simulink model "pi_OfflineRL_H2DF_2023a"  (R2023a)
settings: Solver=FixedStepAuto  StartTime=0.0  StopTime=inf  FixedStep=0.001  RelTol=1e-3  EnableMultiTasking=on
values from neighbouring files (symbols this model uses):
  C2C_NMPC = init_C2C_NMPC_H2DF(C2C_NMPC.expdata)    [init_pi_OfflineRL_H2DF_2023a.m]
  LowerLimit = ([0.17e-3;350;-2;2e-3] - C2C_NMPC.Normalization.controls.mean)./(C2C_NMPC.Normalization.controls.std)    [init_pi_OfflineRL_H2DF_2023a.m]
  UpperLimit = ([0.5e-3;900;10;5.5e-3] - C2C_NMPC.Normalization.controls.mean)./(C2C_NMPC.Normalization.controls.std)    [init_pi_OfflineRL_H2DF_2023a.m]
undefined symbols (not defined in the file or in its folder): DiscIntNeverNeededParam
libraries: deeplib x9, rllib x3, raspberrypiNetworklib x1
(part 2 of 4)

== system pi_OfflineRL_H2DF_2023a/main_C2C_RL/RL_Controller/State_Augmentation ==
  controls : Inport
  Delay1 : Delay  DelayLength=1  InitialCondition=C2C_NMPC.x0(1:C2C_NMPC.Dims.n_LSTM_states)
  Delay3 : Delay  DelayLength=1  InitialCondition=C2C_NMPC.x0
  Delay4 : Delay  DelayLength=1  InitialCondition=C2C_NMPC.x0((C2C_NMPC.Dims.n_states - C2C_NMPC.Dims.n_outputs + 1):C2C_NMPC.Dims.n_states)
  Denorm_plant_IMEP_ref1 : Subsystem
  Display1 : Display
  Mux2 : Mux  Inputs=2
  Mux3 : Mux  Inputs=2
  Selector1 : Selector  IndexOptions=Index vector (dialog)  Indices=[(C2C_NMPC.Dims.n_states - C2C_NMPC.Dims.n_outputs + 1):C2C_NMPC.Dims.n_states]  OutputSizes=1
  Selector3 : Selector  IndexOptions=Index vector (dialog)  Indices=[1]  OutputSizes=1
  dyn_H2DF : Subsystem
  dyn_H2DF_state_augmentation : Subsystem
  LSTM_states : Outport
  wires:
  Delay3/1 -> Selector1/1
  Delay1/1 -> dyn_H2DF/3(last_LSTM_states), dyn_H2DF_state_augmentation/1(last_LSTM_states)
  dyn_H2DF_state_augmentation/1(LSTM_states) -> LSTM_states/1, Delay1/1, Mux3/1
  Mux2/1 -> Mux3/2
  controls/1 -> dyn_H2DF/1(controls), [controls]
  Selector1/1 -> dyn_H2DF/2(last_outputs)
  [controls] -> dyn_H2DF_state_augmentation/2(controls), Mux2/1
  Delay4/1 -> dyn_H2DF_state_augmentation/3(last_outputs)
  Mux3/1 -> Delay3/1
  Denorm_plant_IMEP_ref1/1(RefIn) -> Display1/1
  Selector3/1 -> Denorm_plant_IMEP_ref1/1(outputs)
  dyn_H2DF/1(outputs) -> Selector3/1, Delay4/1, Mux2/2

== system pi_OfflineRL_H2DF_2023a/main_C2C_RL/RL_Controller/Subsystem ==
  note: SOOT
  note: NOX
  note: IMEP
  note: MPRR
  last_outputs : Inport
  Constant : Constant  Value=C2C_NMPC.Normalization.outputs.mean(1)
  Constant1 : Constant  Value=4.8e5
  Constant{4,7,10,12} (4 alike) : Constant  Value=0
  Constant2 : Constant  Value=C2C_NMPC.Normalization.outputs.mean(2)
  Constant3 : Constant  Value=280
  Constant5 : Constant  Value=C2C_NMPC.Normalization.outputs.mean(3)
  Constant6 : Constant  Value=0.1
  Constant8 : Constant  Value=C2C_NMPC.Normalization.outputs.mean(4)
  Constant9 : Constant  Value=5e5
  Demux : Demux
  Gain : Gain  Gain=1/C2C_NMPC.Normalization.outputs.std(1)
  Gain1 : Gain  Gain=1/C2C_NMPC.Normalization.outputs.std(2)
  Gain2 : Gain  Gain=1/C2C_NMPC.Normalization.outputs.std(3)
  Gain3 : Gain  Gain=1/C2C_NMPC.Normalization.outputs.std(4)
  Gain{4..7} (4 alike) : Gain
  Mux : Mux
  Sum{1..3,5} (4 alike) : Sum  Inputs=|+-
  Switch{,1..3} (4 alike) : Switch  Criteria=u2 > Threshold  SaturateOnIntegerOverflow=off  InputSameDT=off
  last_Outputs_Override : Outport
  wires:
  Demux/1 -> Gain4/1
  Constant12/1 -> Switch/2
  last_outputs/1 -> Demux/1
  Constant/1 -> Sum5/2
  Sum5/1 -> Gain/1
  Constant1/1 -> Sum5/1
  Gain/1 -> Switch/1
  Sum1/1 -> Gain1/1
  Constant2/1 -> Sum1/2
  Constant3/1 -> Sum1/1
  Constant4/1 -> Switch1/2
  Gain1/1 -> Switch1/1
  Demux/2 -> Gain5/1
  Switch1/1 -> Mux/2
  Switch2/1 -> Mux/3
  Constant6/1 -> Sum2/1
  Constant5/1 -> Sum2/2
  Sum2/1 -> Gain2/1
  Constant7/1 -> Switch2/2
  Demux/3 -> Gain6/1
  Gain2/1 -> Switch2/1
  Switch3/1 -> Mux/4
  Constant9/1 -> Sum3/1
  Constant8/1 -> Sum3/2
  Sum3/1 -> Gain3/1
  Constant10/1 -> Switch3/2
  Demux/4 -> Gain7/1
  Gain3/1 -> Switch3/1
  Switch/1 -> Mux/1
  Mux/1 -> last_Outputs_Override/1
  Gain4/1 -> Switch/3
  Gain5/1 -> Switch1/3
  Gain6/1 -> Switch2/3
  Gain7/1 -> Switch3/3

== system pi_OfflineRL_H2DF_2023a/main_C2C_RL/RL_Controller/Subsystem1 ==
  In1 : Inport
  If : If  IfExpression=u1 > 4.5e5
  If Action Subsystem : Subsystem  TreatAsAtomicUnit=on
  If Action Subsystem1 : Subsystem  TreatAsAtomicUnit=on
  Merge : Merge
  Out1 : Outport
  wires:
  If Action Subsystem1/1(Out1) -> Merge/2
  If/2 -> If Action Subsystem1/Action
  If/1 -> If Action Subsystem/Action
  In1/1 -> If/1
  Merge/1 -> Out1/1
  If Action Subsystem/1(Out1) -> Merge/1

== system pi_OfflineRL_H2DF_2023a/main_C2C_RL/RL_Controller/dyn_H2DF_state_augmentation ==
  last_LSTM_states : Inport
  controls : Inport  Port=2
  last_outputs : Inport  Port=3
  dyn_H2DF_state_augmentation : MATLAB Function  TreatAsAtomicUnit=on
  LSTM_states : Outport
  wires:
  dyn_H2DF_state_augmentation/1(LSTM_states) -> LSTM_states/1
  last_outputs/1 -> dyn_H2DF_state_augmentation/3(last_outputs)
  last_LSTM_states/1 -> dyn_H2DF_state_augmentation/1(last_LSTM_states)
  controls/1 -> dyn_H2DF_state_augmentation/2(controls)

== system pi_OfflineRL_H2DF_2023a/main_C2C_RL/post_processing/ denormalizing reference ==
  IMEP_norm : Inport
  NOX_norm : Inport  Port=2
  soot_norm : Inport  Port=3
  MPRR_norm : Inport  Port=4
  Constant : Constant  Value=C2C_NMPC.Normalization.outputs.mean(1)
  Constant1 : Constant  Value=C2C_NMPC.Normalization.outputs.mean(2)
  Constant2 : Constant  Value=C2C_NMPC.Normalization.outputs.mean(3)
  Constant3 : Constant  Value=C2C_NMPC.Normalization.outputs.mean(4)
  Gain : Gain  Gain=C2C_NMPC.Normalization.outputs.std(1)
  Gain1 : Gain  Gain=C2C_NMPC.Normalization.outputs.std(2)
  Gain2 : Gain  Gain=C2C_NMPC.Normalization.outputs.std(3)
  Gain3 : Gain  Gain=C2C_NMPC.Normalization.outputs.std(4)
  Sum{1..3,5} (4 alike) : Sum  Inputs=|++
  IMEP : Outport
  NOX : Outport  Port=2
  soot : Outport  Port=3
  MPRR : Outport  Port=4
  wires:
  Gain/1 -> Sum5/1
  IMEP_norm/1 -> Gain/1
  Constant/1 -> Sum5/2
  Sum5/1 -> IMEP/1
  Gain1/1 -> Sum1/1
  Constant1/1 -> Sum1/2
  NOX_norm/1 -> Gain1/1
  Sum1/1 -> NOX/1
  Gain2/1 -> Sum2/1
  Constant2/1 -> Sum2/2
  soot_norm/1 -> Gain2/1
  Sum2/1 -> soot/1
  Gain3/1 -> Sum3/1
  Constant3/1 -> Sum3/2
  MPRR_norm/1 -> Gain3/1
  Sum3/1 -> MPRR/1

== system pi_OfflineRL_H2DF_2023a/main_C2C_RL/post_processing/Subsystem ==
  controller_ status : Inport
  LSTM_States : Inport  Port=2
  Selector2 : Selector  IndexOptions=Index vector (dialog)  Indices=[1:(C2C_NMPC.Dims.n_hidden_states+ C2C_NMPC.Dims.n_cell_states)]  OutputSizes=1
  Selector3 : Selector  IndexOptions=Index vector (dialog)  Indices=[41:56]  OutputSizes=1
  Subtract : Sum  Inputs=+-
  Out1 : Outport
  wires:
  Selector3/1 -> Subtract/1
  Selector2/1 -> Subtract/2
  controller_ status/1 -> Selector3/1
  Subtract/1 -> Out1/1
  LSTM_States/1 -> Selector2/1

== system pi_OfflineRL_H2DF_2023a/main_C2C_RL/post_processing/Subsystem1 ==
  controller_ status : Inport
  Last_Output_MC : Inport  Port=2
  " denormalizing reference" : Subsystem
  Demux : Demux
  Mux : Mux
  Mux1 : Mux  Inputs=2
  Mux2 : Mux
  Selector1 : Selector  IndexOptions=Index vector (dialog)  Indices=[(4 + C2C_NMPC.Dims.n_controls * C2C_NMPC.Opts.N + 1 * (C2C_NMPC.Dims.n_states) + C2C_NMPC.Dims.n_LSTM_states + C2C_NMPC.Dims.n_controls +1):( 4 + C2C_NMPC.Dims.n_controls * C2C_NMPC.Opts.N + 2* C2C_NMPC.Dims.n_states)]  OutputSizes=1
  Selector2 : Selector  IndexOptions=Index vector (dialog)  Indices=[(4 + C2C_NMPC.Dims.n_controls * C2C_NMPC.Opts.N + 2 * (C2C_NMPC.Dims.n_states) + C2C_NMPC.Dims.n_LSTM_states + C2C_NMPC.Dims.n_controls +1):( 4 + C2C_NMPC.Dims.n_controls * C2C_NMPC.Opts.N + 3* C2C_NMPC.Dims.n_states)]  OutputSizes=1
  Selector3 : Selector  IndexOptions=Index vector (dialog)  Indices=[(4 + C2C_NMPC.Dims.n_controls * C2C_NMPC.Opts.N + 1* (C2C_NMPC.Dims.n_LSTM_states + C2C_NMPC.Dims.n_controls) +1) : (4 + C2C_NMPC.Dims.n_controls * C2C_NMPC.Opts.N + 1* C2C_NMPC.Dims.n_states)]  OutputSizes=1
  Selector4 : Selector  IndexOptions=Index vector (dialog)  Indices=[(4 + C2C_NMPC.Dims.n_controls * C2C_NMPC.Opts.N + 3 * (C2C_NMPC.Dims.n_states) + C2C_NMPC.Dims.n_LSTM_states + C2C_NMPC.Dims.n_controls +1):( 4 + C2C_NMPC.Dims.n_controls * C2C_NMPC.Opts.N + 4* C2C_NMPC.Dims.n_states)]  OutputSizes=1
  Subsystem : Subsystem
  Out1 : Outport
  wires:
  Last_Output_MC/1 -> Demux/1
  controller_ status/1 -> Selector4/1, Selector2/1, Selector1/1, Selector3/1
  Mux1/1 -> Out1/1
  Mux/1 -> Mux1/2
  Demux/1 -> " denormalizing reference"/1(IMEP_norm)
  Demux/2 -> " denormalizing reference"/2(NOX_norm)
  Demux/3 -> " denormalizing reference"/3(soot_norm)
  Demux/4 -> " denormalizing reference"/4(MPRR_norm)
  " denormalizing reference"/2(NOX) -> Mux2/2
  " denormalizing reference"/1(IMEP) -> Mux2/1
  " denormalizing reference"/3(soot) -> Mux2/3
  " denormalizing reference"/4(MPRR) -> Mux2/4
  Mux2/1 -> Mux1/1
  Subsystem/1(Node_0) -> Mux/1
  Selector3/1 -> Subsystem/1(In1)
  Selector1/1 -> Subsystem/2(In2)
  Subsystem/2(Node_1) -> Mux/2
  Subsystem/3(Node_2) -> Mux/3
  Subsystem/4(Node_3) -> Mux/4
  Selector4/1 -> Subsystem/4(In4)
  Selector2/1 -> Subsystem/3(In3)

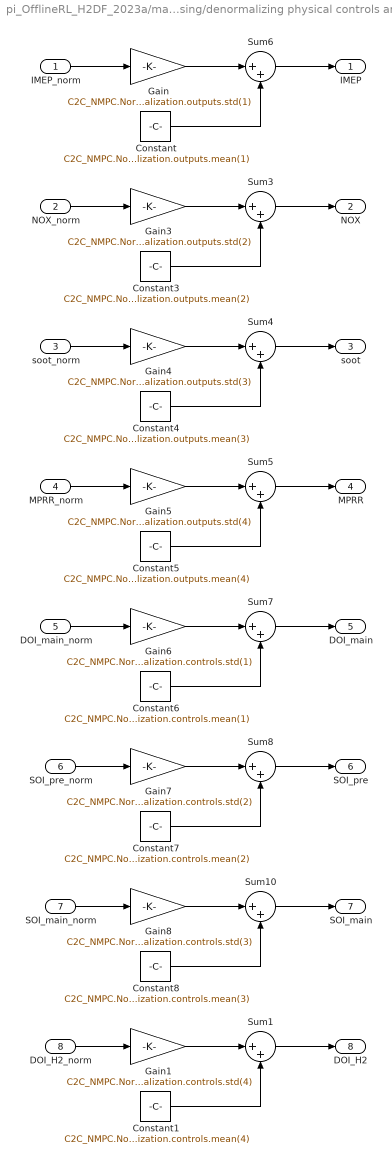
== system pi_OfflineRL_H2DF_2023a/main_C2C_RL/post_processing/denormalizing physical controls and outputs ==
  IMEP_norm : Inport
  NOX_norm : Inport  Port=2
  soot_norm : Inport  Port=3
  MPRR_norm : Inport  Port=4
  DOI_main_norm : Inport  Port=5
  SOI_pre_norm : Inport  Port=6
  SOI_main_norm : Inport  Port=7
  DOI_H2_norm : Inport  Port=8
  Constant : Constant  Value=C2C_NMPC.Normalization.outputs.mean(1)
  Constant1 : Constant  Value=C2C_NMPC.Normalization.controls.mean(4)
  Constant3 : Constant  Value=C2C_NMPC.Normalization.outputs.mean(2)
  Constant4 : Constant  Value=C2C_NMPC.Normalization.outputs.mean(3)
  Constant5 : Constant  Value=C2C_NMPC.Normalization.outputs.mean(4)
  Constant6 : Constant  Value=C2C_NMPC.Normalization.controls.mean(1)
  Constant7 : Constant  Value=C2C_NMPC.Normalization.controls.mean(2)
  Constant8 : Constant  Value=C2C_NMPC.Normalization.controls.mean(3)
  Gain : Gain  Gain=C2C_NMPC.Normalization.outputs.std(1)
  Gain1 : Gain  Gain=C2C_NMPC.Normalization.controls.std(4)
  Gain3 : Gain  Gain=C2C_NMPC.Normalization.outputs.std(2)
  Gain4 : Gain  Gain=C2C_NMPC.Normalization.outputs.std(3)
  Gain5 : Gain  Gain=C2C_NMPC.Normalization.outputs.std(4)
  Gain6 : Gain  Gain=C2C_NMPC.Normalization.controls.std(1)
  Gain7 : Gain  Gain=C2C_NMPC.Normalization.controls.std(2)
  Gain8 : Gain  Gain=C2C_NMPC.Normalization.controls.std(3)
  Sum{1,3..8,10} (8 alike) : Sum  Inputs=|++
  IMEP : Outport
  NOX : Outport  Port=2
  soot : Outport  Port=3
  MPRR : Outport  Port=4
  DOI_main : Outport  Port=5
  SOI_pre : Outport  Port=6
  SOI_main : Outport  Port=7
  DOI_H2 : Outport  Port=8
  wires:
  Gain4/1 -> Sum4/1
  Constant3/1 -> Sum3/2
  Constant4/1 -> Sum4/2
  Gain3/1 -> Sum3/1
  Constant5/1 -> Sum5/2
  Gain5/1 -> Sum5/1
  Constant/1 -> Sum6/2
  Sum3/1 -> NOX/1
  NOX_norm/1 -> Gain3/1
  Sum5/1 -> MPRR/1
  Gain/1 -> Sum6/1
  IMEP_norm/1 -> Gain/1
  Sum6/1 -> IMEP/1
  MPRR_norm/1 -> Gain5/1
  Sum4/1 -> soot/1
  soot_norm/1 -> Gain4/1
  Constant7/1 -> Sum8/2
  Gain8/1 -> Sum10/1
  Constant6/1 -> Sum7/2
  Gain7/1 -> Sum8/1
  Sum10/1 -> SOI_main/1
  DOI_main_norm/1 -> Gain6/1
  Sum7/1 -> DOI_main/1
  Gain6/1 -> Sum7/1
  Sum8/1 -> SOI_pre/1
  Constant8/1 -> Sum10/2
  SOI_main_norm/1 -> Gain8/1
  SOI_pre_norm/1 -> Gain7/1
  Sum1/1 -> DOI_H2/1
  Constant1/1 -> Sum1/2
  Gain1/1 -> Sum1/1
  DOI_H2_norm/1 -> Gain1/1

== system pi_OfflineRL_H2DF_2023a/main_C2C_RL/pre_processing1/normalize_last_outputs_MC ==
  data_in : Inport
  Constant : Constant  Value=C2C_NMPC.Normalization.outputs.mean(1)
  Constant1 : Constant  Value=C2C_NMPC.Normalization.outputs.mean(2)
  Constant2 : Constant  Value=C2C_NMPC.Normalization.outputs.mean(3)
  Constant3 : Constant  Value=C2C_NMPC.Normalization.outputs.mean(4)
  Demux : Demux
  Gain : Gain  Gain=1/C2C_NMPC.Normalization.outputs.std(1)
  Gain1 : Gain  Gain=1/C2C_NMPC.Normalization.outputs.std(2)
  Gain2 : Gain  Gain=1/C2C_NMPC.Normalization.outputs.std(3)
  Gain3 : Gain  Gain=1/C2C_NMPC.Normalization.outputs.std(4)
  Mux : Mux
  Selector1 : Selector  IndexOptions=Index vector (dialog)  Indices=[1:4]  OutputSizes=1
  Sum{1..3,5} (4 alike) : Sum  Inputs=|+-
  last_outputs_MC : Outport  VectorParamsAs1DForOutWhenUnconnected=off
  wires:
  Demux/2 -> Sum1/1
  Constant2/1 -> Sum2/2
  Sum2/1 -> Gain2/1
  Sum1/1 -> Gain1/1
  Gain3/1 -> Mux/4
  Gain1/1 -> Mux/2
  Constant1/1 -> Sum1/2
  Demux/3 -> Sum2/1
  Gain2/1 -> Mux/3
  Mux/1 -> last_outputs_MC/1
  Constant3/1 -> Sum3/2
  Sum3/1 -> Gain3/1
  Gain/1 -> Mux/1
  Sum5/1 -> Gain/1
  Constant/1 -> Sum5/2
  Demux/1 -> Sum5/1
  data_in/1 -> Selector1/1
  Demux/4 -> Sum3/1
  Selector1/1 -> Demux/1

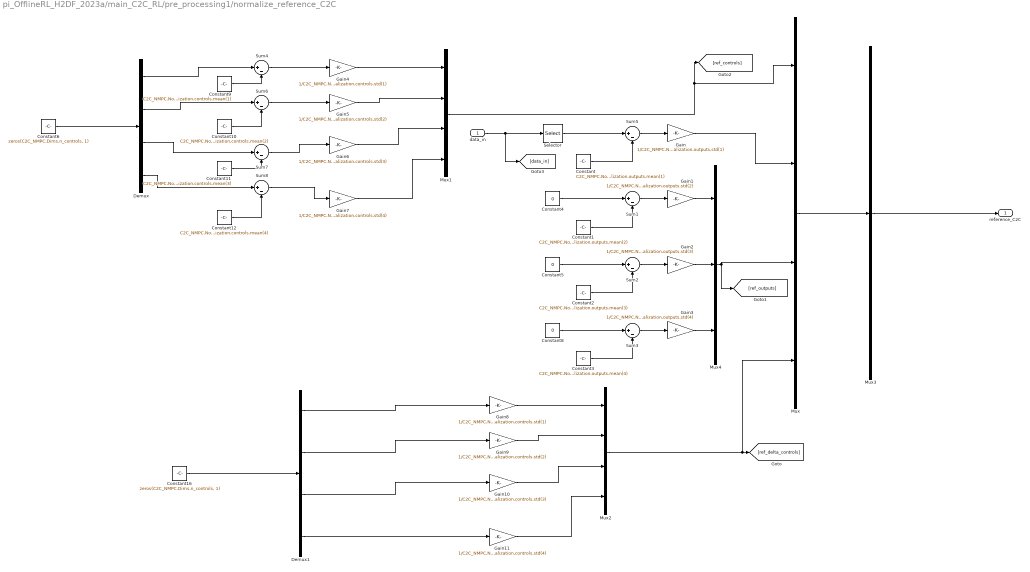
== system pi_OfflineRL_H2DF_2023a/main_C2C_RL/pre_processing1/normalize_reference_C2C ==
  data_in : Inport
  Constant : Constant  Value=C2C_NMPC.Normalization.outputs.mean(1)
  Constant1 : Constant  Value=C2C_NMPC.Normalization.outputs.mean(2)
  Constant10 : Constant  Value=C2C_NMPC.Normalization.controls.mean(2)
  Constant11 : Constant  Value=C2C_NMPC.Normalization.controls.mean(3)
  Constant12 : Constant  Value=C2C_NMPC.Normalization.controls.mean(4)
  Constant16 : Constant  Value=zeros(C2C_NMPC.Dims.n_controls, 1)
  Constant2 : Constant  Value=C2C_NMPC.Normalization.outputs.mean(3)
  Constant3 : Constant  Value=C2C_NMPC.Normalization.outputs.mean(4)
  Constant4 : Constant  Value=0
  Constant5 : Constant  Value=0
  Constant6 : Constant  Value=zeros(C2C_NMPC.Dims.n_controls, 1)
  Constant8 : Constant  Value=0
  Constant9 : Constant  Value=C2C_NMPC.Normalization.controls.mean(1)
  Demux : Demux
  Demux1 : Demux
  Gain : Gain  Gain=1/C2C_NMPC.Normalization.outputs.std(1)
  Gain1 : Gain  Gain=1/C2C_NMPC.Normalization.outputs.std(2)
  Gain10 : Gain  Gain=1/C2C_NMPC.Normalization.controls.std(3)
  Gain11 : Gain  Gain=1/C2C_NMPC.Normalization.controls.std(4)
  Gain2 : Gain  Gain=1/C2C_NMPC.Normalization.outputs.std(3)
  Gain3 : Gain  Gain=1/C2C_NMPC.Normalization.outputs.std(4)
  Gain4 : Gain  Gain=1/C2C_NMPC.Normalization.controls.std(1)
  Gain5 : Gain  Gain=1/C2C_NMPC.Normalization.controls.std(2)
  Gain6 : Gain  Gain=1/C2C_NMPC.Normalization.controls.std(3)
  Gain7 : Gain  Gain=1/C2C_NMPC.Normalization.controls.std(4)
  Gain8 : Gain  Gain=1/C2C_NMPC.Normalization.controls.std(1)
  Gain9 : Gain  Gain=1/C2C_NMPC.Normalization.controls.std(2)
  Mux : Mux
  Mux1 : Mux
  Mux2 : Mux
  Mux3 : Mux  Inputs=1
  Mux4 : Mux  Inputs=3
  Selector : Selector  IndexOptions=Index vector (dialog)  Indices=[5]  OutputSizes=1
  Sum{1..8} (8 alike) : Sum  Inputs=|+-
  reference_C2C : Outport  VectorParamsAs1DForOutWhenUnconnected=off
  wires:
  Constant/1 -> Sum5/2
  data_in/1 -> [data_in], Selector/1
  Sum5/1 -> Gain/1
  Selector/1 -> Sum5/1
  Constant4/1 -> Sum1/1
  Sum1/1 -> Gain1/1
  Constant1/1 -> Sum1/2
  Constant5/1 -> Sum2/1
  Sum2/1 -> Gain2/1
  Constant2/1 -> Sum2/2
  Constant8/1 -> Sum3/1
  Sum3/1 -> Gain3/1
  Constant3/1 -> Sum3/2
  Demux/1 -> Sum4/1
  Sum4/1 -> Gain4/1
  Constant9/1 -> Sum4/2
  Constant6/1 -> Demux/1
  Demux/2 -> Sum6/1
  Constant10/1 -> Sum6/2
  Sum6/1 -> Gain5/1
  Gain5/1 -> Mux1/2
  Gain4/1 -> Mux1/1
  Sum7/1 -> Gain6/1
  Constant11/1 -> Sum7/2
  Demux/3 -> Sum7/1
  Constant12/1 -> Sum8/2
  Sum8/1 -> Gain7/1
  Demux/4 -> Sum8/1
  Gain7/1 -> Mux1/4
  Gain6/1 -> Mux1/3
  Gain9/1 -> Mux2/2
  Gain11/1 -> Mux2/4
  Constant16/1 -> Demux1/1
  Gain8/1 -> Mux2/1
  Gain10/1 -> Mux2/3
  Demux1/4 -> Gain11/1
  Demux1/3 -> Gain10/1
  Demux1/2 -> Gain9/1
  Demux1/1 -> Gain8/1
  Mux2/1 -> [ref_delta_controls], Mux/4
  Mux3/1 -> reference_C2C/1
  Mux/1 -> Mux3/1
  Gain1/1 -> Mux4/1
  Gain2/1 -> Mux4/2
  Gain3/1 -> Mux4/3
  Gain/1 -> Mux/2
  Mux4/1 -> Mux/3, [ref_outputs]
  Mux1/1 -> [ref_controls], Mux/1

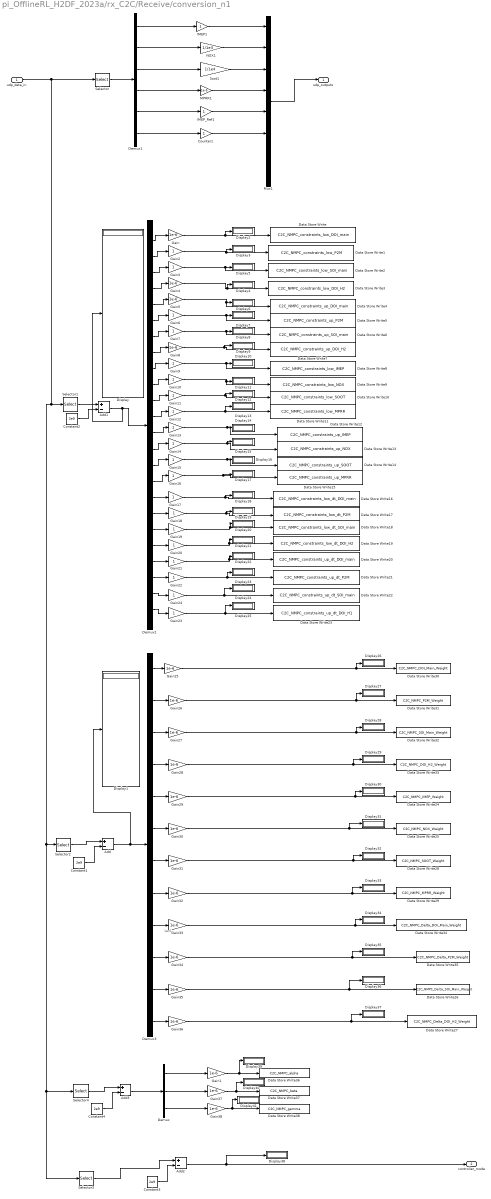
== system pi_OfflineRL_H2DF_2023a/rx_C2C/Receive/conversion_n1 ==
  note: 1e-6
  udp_data_in : Inport
  Add{,1..3} (4 alike) : Sum  Inputs=+-
  Constant{1..4} (4 alike) : Constant  Value=2e9
  Counter1 : Gain
  Data Store Write : DataStoreWrite  DataStoreName=C2C_NMPC_constraints_low_DOI_main  IndexOptions=Index vector (dialog)  Indices=1  OutputSizes=1
  Data Store Write1 : DataStoreWrite  DataStoreName=C2C_NMPC_constraints_low_P2M  IndexOptions=Index vector (dialog)  Indices=1  OutputSizes=1
  Data Store Write10 : DataStoreWrite  DataStoreName=C2C_NMPC_constraints_low_SOOT  IndexOptions=Index vector (dialog)  Indices=1  OutputSizes=1
  Data Store Write11 : DataStoreWrite  DataStoreName=C2C_NMPC_constraints_low_MPRR  IndexOptions=Index vector (dialog)  Indices=1  OutputSizes=1
  Data Store Write12 : DataStoreWrite  DataStoreName=C2C_NMPC_constraints_up_IMEP  IndexOptions=Index vector (dialog)  Indices=1  OutputSizes=1
  Data Store Write13 : DataStoreWrite  DataStoreName=C2C_NMPC_constraints_up_NOX  IndexOptions=Index vector (dialog)  Indices=1  OutputSizes=1
  Data Store Write14 : DataStoreWrite  DataStoreName=C2C_NMPC_constraints_up_SOOT  IndexOptions=Index vector (dialog)  Indices=1  OutputSizes=1
  Data Store Write15 : DataStoreWrite  DataStoreName=C2C_NMPC_constraints_up_MPRR  IndexOptions=Index vector (dialog)  Indices=1  OutputSizes=1
  Data Store Write16 : DataStoreWrite  DataStoreName=C2C_NMPC_constraints_low_dt_DOI_main  IndexOptions=Index vector (dialog)  Indices=1  OutputSizes=1
  Data Store Write17 : DataStoreWrite  DataStoreName=C2C_NMPC_constraints_low_dt_P2M  IndexOptions=Index vector (dialog)  Indices=1  OutputSizes=1
  Data Store Write18 : DataStoreWrite  DataStoreName=C2C_NMPC_constraints_low_dt_SOI_main  IndexOptions=Index vector (dialog)  Indices=1  OutputSizes=1
  Data Store Write19 : DataStoreWrite  DataStoreName=C2C_NMPC_constraints_low_dt_DOI_H2  IndexOptions=Index vector (dialog)  Indices=1  OutputSizes=1
  Data Store Write2 : DataStoreWrite  DataStoreName=C2C_NMPC_constraints_low_SOI_main  IndexOptions=Index vector (dialog)  Indices=1  OutputSizes=1
  Data Store Write20 : DataStoreWrite  DataStoreName=C2C_NMPC_constraints_up_dt_DOI_main  IndexOptions=Index vector (dialog)  Indices=1  OutputSizes=1
  Data Store Write21 : DataStoreWrite  DataStoreName=C2C_NMPC_constraints_up_dt_P2M  IndexOptions=Index vector (dialog)  Indices=1  OutputSizes=1
  Data Store Write22 : DataStoreWrite  DataStoreName=C2C_NMPC_constraints_up_dt_SOI_main  IndexOptions=Index vector (dialog)  Indices=1  OutputSizes=1
  Data Store Write23 : DataStoreWrite  DataStoreName=C2C_NMPC_constraints_up_dt_DOI_H1  IndexOptions=Index vector (dialog)  Indices=1  OutputSizes=1
  Data Store Write24 : DataStoreWrite  DataStoreName=C2C_NMPC_IMEP_Weight  IndexOptions=Index vector (dialog)  Indices=1  OutputSizes=1
  Data Store Write25 : DataStoreWrite  DataStoreName=C2C_NMPC_NOX_Weight  IndexOptions=Index vector (dialog)  Indices=1  OutputSizes=1
  Data Store Write26 : DataStoreWrite  DataStoreName=C2C_NMPC_Delta_SOI_Main_Weight  IndexOptions=Index vector (dialog)  Indices=1  OutputSizes=1
  Data Store Write27 : DataStoreWrite  DataStoreName=C2C_NMPC_Delta_DOI_H2_Weight  IndexOptions=Index vector (dialog)  Indices=1  OutputSizes=1
  Data Store Write28 : DataStoreWrite  DataStoreName=C2C_NMPC_SOOT_Weight  IndexOptions=Index vector (dialog)  Indices=1  OutputSizes=1
  Data Store Write29 : DataStoreWrite  DataStoreName=C2C_NMPC_MPRR_Weight  IndexOptions=Index vector (dialog)  Indices=1  OutputSizes=1
  Data Store Write3 : DataStoreWrite  DataStoreName=C2C_NMPC_constraints_low_DOI_H2  IndexOptions=Index vector (dialog)  Indices=1  OutputSizes=1
  Data Store Write30 : DataStoreWrite  DataStoreName=C2C_NMPC_DOI_Main_Weight  IndexOptions=Index vector (dialog)  Indices=1  OutputSizes=1
  Data Store Write31 : DataStoreWrite  DataStoreName=C2C_NMPC_P2M_Weight  IndexOptions=Index vector (dialog)  Indices=1  OutputSizes=1
  Data Store Write32 : DataStoreWrite  DataStoreName=C2C_NMPC_SOI_Main_Weight  IndexOptions=Index vector (dialog)  Indices=1  OutputSizes=1
  Data Store Write33 : DataStoreWrite  DataStoreName=C2C_NMPC_DOI_H2_Weight  IndexOptions=Index vector (dialog)  Indices=1  OutputSizes=1
  Data Store Write34 : DataStoreWrite  DataStoreName=C2C_NMPC_Delta_DOI_Main_Weight  IndexOptions=Index vector (dialog)  Indices=1  OutputSizes=1
  Data Store Write35 : DataStoreWrite  DataStoreName=C2C_NMPC_Delta_P2M_Weight  IndexOptions=Index vector (dialog)  Indices=1  OutputSizes=1
  Data Store Write36 : DataStoreWrite  DataStoreName=C2C_NMPC_alpha  IndexOptions=Index vector (dialog)  Indices=1  OutputSizes=1
  Data Store Write37 : DataStoreWrite  DataStoreName=C2C_NMPC_beta  IndexOptions=Index vector (dialog)  Indices=1  OutputSizes=1
  Data Store Write38 : DataStoreWrite  DataStoreName=C2C_NMPC_gamma  IndexOptions=Index vector (dialog)  Indices=1  OutputSizes=1
  Data Store Write4 : DataStoreWrite  DataStoreName=C2C_NMPC_constraints_up_DOI_main  IndexOptions=Index vector (dialog)  Indices=1  OutputSizes=1
  Data Store Write5 : DataStoreWrite  DataStoreName=C2C_NMPC_constraints_up_P2M  IndexOptions=Index vector (dialog)  Indices=1  OutputSizes=1
  Data Store Write6 : DataStoreWrite  DataStoreName=C2C_NMPC_constraints_up_SOI_main  IndexOptions=Index vector (dialog)  Indices=1  OutputSizes=1
  Data Store Write7 : DataStoreWrite  DataStoreName=C2C_NMPC_constraints_up_DOI_H2  IndexOptions=Index vector (dialog)  Indices=1  OutputSizes=1
  Data Store Write8 : DataStoreWrite  DataStoreName=C2C_NMPC_constraints_low_IMEP  IndexOptions=Index vector (dialog)  Indices=1  OutputSizes=1
  Data Store Write9 : DataStoreWrite  DataStoreName=C2C_NMPC_constraints_low_NOX  IndexOptions=Index vector (dialog)  Indices=1  OutputSizes=1
  Demux : Demux  Outputs=3
  Demux1 : Demux  Outputs=6
  Demux2 : Demux  Outputs=24
  Demux3 : Demux  Outputs=12
  Display{,1..41} (42 alike) : Display
  Gain{,1,4..5,8,25..38} (19 alike) : Gain  Gain=1e-6
  Gain{2..3,6..7,9..24} (20 alike) : Gain
  IMEP1 : Gain
  IMEP_Ref1 : Gain
  MPRR1 : Gain  Gain=1e-5
  Mux1 : Mux  Inputs=8
  NOX1 : Gain  Gain=1/1e3
  Selector : Selector  IndexOptions=Index vector (dialog)  Indices=[1:6]  OutputSizes=1
  Selector1 : Selector  IndexOptions=Index vector (dialog)  Indices=[7:30]  OutputSizes=1
  Selector2 : Selector  IndexOptions=Index vector (dialog)  Indices=[31:42]  OutputSizes=1
  Selector3 : Selector  IndexOptions=Index vector (dialog)  Indices=[46]  OutputSizes=1
  Selector4 : Selector  IndexOptions=Index vector (dialog)  Indices=[43:45]  OutputSizes=1
  Soot1 : Gain  Gain=1/1e4
  udp_outputs : Outport
  controller_mode : Outport  Port=2
  wires:
  Gain38/1 -> Data Store Write38/1, Display41/1
  Gain1/1 -> Data Store Write36/1, Display39/1
  Gain37/1 -> Data Store Write37/1, Display40/1
  Demux/3 -> Gain38/1
  Demux/2 -> Gain37/1
  Demux/1 -> Gain1/1
  Add3/1 -> Demux/1
  Selector4/1 -> Add3/1
  Constant4/1 -> Add3/2
  Add2/1 -> Display38/1, controller_mode/1
  Selector3/1 -> Add2/1
  Constant3/1 -> Add2/2
  Constant2/1 -> Add1/2
  Add1/1 -> Demux2/1, Display/1
  Selector1/1 -> Add1/1
  Selector2/1 -> Add/1
  Gain36/1 -> Data Store Write27/1, Display37/1
  Gain35/1 -> Data Store Write26/1, Display36/1
  Gain34/1 -> Data Store Write35/1, Display35/1
  Gain33/1 -> Data Store Write34/1, Display34/1
  Gain32/1 -> Data Store Write29/1, Display33/1
  Gain31/1 -> Data Store Write28/1, Display32/1
  Gain30/1 -> Data Store Write25/1, Display31/1
  Gain29/1 -> Data Store Write24/1, Display30/1
  Gain28/1 -> Data Store Write33/1, Display29/1
  Gain27/1 -> Data Store Write32/1, Display28/1
  Gain26/1 -> Data Store Write31/1, Display27/1
  Gain25/1 -> Data Store Write30/1, Display26/1
  Gain24/1 -> Data Store Write22/1, Display24/1
  Gain23/1 -> Data Store Write23/1, Display25/1
  Gain22/1 -> Data Store Write21/1, Display23/1
  Gain21/1 -> Data Store Write20/1, Display22/1
  Gain20/1 -> Data Store Write19/1, Display21/1
  Gain19/1 -> Data Store Write18/1, Display20/1
  Gain18/1 -> Data Store Write17/1, Display19/1
  Gain17/1 -> Data Store Write16/1, Display18/1
  Gain16/1 -> Data Store Write15/1, Display17/1
  Gain15/1 -> Display16/1, Data Store Write14/1
  Gain14/1 -> Data Store Write13/1, Display15/1
  Gain13/1 -> Display14/1, Data Store Write12/1
  Gain12/1 -> Data Store Write11/1, Display13/1
  Gain11/1 -> Data Store Write10/1, Display12/1
  Gain10/1 -> Data Store Write9/1, Display11/1
  Gain9/1 -> Data Store Write8/1, Display10/1
  Gain8/1 -> Data Store Write7/1, Display9/1
  Gain7/1 -> Data Store Write6/1, Display8/1
  Gain6/1 -> Data Store Write5/1, Display7/1
  Gain5/1 -> Data Store Write4/1, Display6/1
  Gain4/1 -> Data Store Write3/1, Display4/1
  Gain3/1 -> Display5/1, Data Store Write2/1
  Gain2/1 -> Data Store Write1/1, Display3/1
  Gain/1 -> Data Store Write/1, Display2/1
  Constant1/1 -> Add/2
  Add/1 -> Demux3/1, Display1/1
  Demux3/5 -> Gain29/1
  IMEP1/1 -> Mux1/1
  Demux1/5 -> IMEP_Ref1/1
  Demux3/12 -> Gain36/1
  Soot1/1 -> Mux1/3
  NOX1/1 -> Mux1/2
  udp_data_in/1 -> Selector/1, Selector1/1, Selector2/1, Selector4/1, Selector3/1
  Counter1/1 -> Mux1/6
  Demux1/6 -> Counter1/1
  Demux3/1 -> Gain25/1
  Demux3/7 -> Gain31/1
  Demux1/4 -> MPRR1/1
  Demux3/4 -> Gain28/1
  Demux2/8 -> Gain8/1
  Demux2/24 -> Gain23/1
  Demux2/17 -> Gain17/1
  Mux1/1 -> udp_outputs/1
  Demux2/6 -> Gain6/1
  Demux3/6 -> Gain30/1
  Selector/1 -> Demux1/1
  Demux2/5 -> Gain5/1
  Demux2/11 -> Gain11/1
  Demux2/20 -> Gain20/1
  Demux2/14 -> Gain14/1
  Demux2/13 -> Gain13/1
  Demux2/22 -> Gain22/1
  Demux2/4 -> Gain4/1
  Demux3/8 -> Gain32/1
  Demux2/10 -> Gain10/1
  Demux3/10 -> Gain34/1
  Demux2/7 -> Gain7/1
  Demux2/15 -> Gain15/1
  Demux3/3 -> Gain27/1
  Demux1/3 -> Soot1/1
  MPRR1/1 -> Mux1/4
  Demux2/21 -> Gain21/1
  Demux2/19 -> Gain19/1
  Demux2/12 -> Gain12/1
  Demux1/2 -> NOX1/1
  Demux3/2 -> Gain26/1
  Demux2/18 -> Gain18/1
  Demux2/23 -> Gain24/1
  Demux2/3 -> Gain3/1
  Demux1/1 -> IMEP1/1
  Demux3/11 -> Gain35/1
  Demux2/2 -> Gain2/1
  Demux2/9 -> Gain9/1
  IMEP_Ref1/1 -> Mux1/5
  Demux3/9 -> Gain33/1
  Demux2/1 -> Gain/1
  Demux2/16 -> Gain16/1

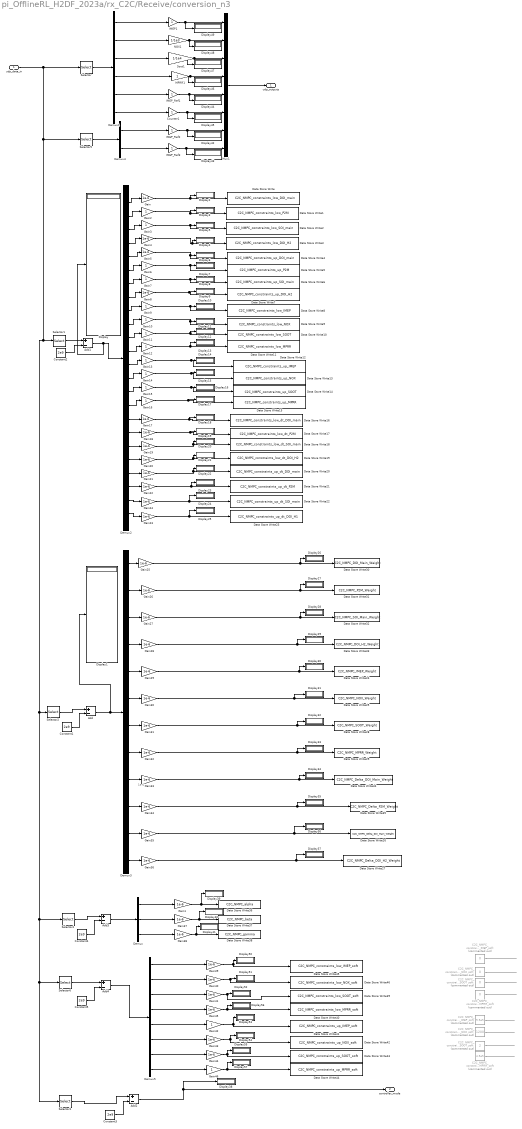
== system pi_OfflineRL_H2DF_2023a/rx_C2C/Receive/conversion_n3 ==
  note: 1e-6
  udp_data_in : Inport
  Add{,1..4} (5 alike) : Sum  Inputs=+-
  C2C_NMPC_constraints_low_IMEP_soft : Constant  Commented=on  Value=0
  C2C_NMPC_constraints_low_MPRR_soft : Constant  Commented=on  Value=0
  C2C_NMPC_constraints_low_NOX_soft : Constant  Commented=on  Value=0
  C2C_NMPC_constraints_low_SOOT_soft : Constant  Commented=on  Value=0
  C2C_NMPC_constraints_up_IMEP_soft : Constant  Commented=on  Value=9.5e5
  C2C_NMPC_constraints_up_MPRR_soft : Constant  Commented=on  Value=4.5e5
  C2C_NMPC_constraints_up_NOX_soft : Constant  Commented=on  Value=1200
  C2C_NMPC_constraints_up_SOOT_soft : Constant  Commented=on  Value=2
  Constant{1..5} (5 alike) : Constant  Value=2e9
  Counter1 : Gain
  Data Store Write : DataStoreWrite  DataStoreName=C2C_NMPC_constraints_low_DOI_main  IndexOptions=Index vector (dialog)  Indices=1  OutputSizes=1
  Data Store Write1 : DataStoreWrite  DataStoreName=C2C_NMPC_constraints_low_P2M  IndexOptions=Index vector (dialog)  Indices=1  OutputSizes=1
  Data Store Write10 : DataStoreWrite  DataStoreName=C2C_NMPC_constraints_low_SOOT  IndexOptions=Index vector (dialog)  Indices=1  OutputSizes=1
  Data Store Write11 : DataStoreWrite  DataStoreName=C2C_NMPC_constraints_low_MPRR  IndexOptions=Index vector (dialog)  Indices=1  OutputSizes=1
  Data Store Write12 : DataStoreWrite  DataStoreName=C2C_NMPC_constraints_up_IMEP  IndexOptions=Index vector (dialog)  Indices=1  OutputSizes=1
  Data Store Write13 : DataStoreWrite  DataStoreName=C2C_NMPC_constraints_up_NOX  IndexOptions=Index vector (dialog)  Indices=1  OutputSizes=1
  Data Store Write14 : DataStoreWrite  DataStoreName=C2C_NMPC_constraints_up_SOOT  IndexOptions=Index vector (dialog)  Indices=1  OutputSizes=1
  Data Store Write15 : DataStoreWrite  DataStoreName=C2C_NMPC_constraints_up_MPRR  IndexOptions=Index vector (dialog)  Indices=1  OutputSizes=1
  Data Store Write16 : DataStoreWrite  DataStoreName=C2C_NMPC_constraints_low_dt_DOI_main  IndexOptions=Index vector (dialog)  Indices=1  OutputSizes=1
  Data Store Write17 : DataStoreWrite  DataStoreName=C2C_NMPC_constraints_low_dt_P2M  IndexOptions=Index vector (dialog)  Indices=1  OutputSizes=1
  Data Store Write18 : DataStoreWrite  DataStoreName=C2C_NMPC_constraints_low_dt_SOI_main  IndexOptions=Index vector (dialog)  Indices=1  OutputSizes=1
  Data Store Write19 : DataStoreWrite  DataStoreName=C2C_NMPC_constraints_low_dt_DOI_H2  IndexOptions=Index vector (dialog)  Indices=1  OutputSizes=1
  Data Store Write2 : DataStoreWrite  DataStoreName=C2C_NMPC_constraints_low_SOI_main  IndexOptions=Index vector (dialog)  Indices=1  OutputSizes=1
  Data Store Write20 : DataStoreWrite  DataStoreName=C2C_NMPC_constraints_up_dt_DOI_main  IndexOptions=Index vector (dialog)  Indices=1  OutputSizes=1
  Data Store Write21 : DataStoreWrite  DataStoreName=C2C_NMPC_constraints_up_dt_P2M  IndexOptions=Index vector (dialog)  Indices=1  OutputSizes=1
  Data Store Write22 : DataStoreWrite  DataStoreName=C2C_NMPC_constraints_up_dt_SOI_main  IndexOptions=Index vector (dialog)  Indices=1  OutputSizes=1
  Data Store Write23 : DataStoreWrite  DataStoreName=C2C_NMPC_constraints_up_dt_DOI_H1  IndexOptions=Index vector (dialog)  Indices=1  OutputSizes=1
  Data Store Write24 : DataStoreWrite  DataStoreName=C2C_NMPC_IMEP_Weight  IndexOptions=Index vector (dialog)  Indices=1  OutputSizes=1
  Data Store Write25 : DataStoreWrite  DataStoreName=C2C_NMPC_NOX_Weight  IndexOptions=Index vector (dialog)  Indices=1  OutputSizes=1
  Data Store Write26 : DataStoreWrite  DataStoreName=C2C_NMPC_Delta_SOI_Main_Weight  IndexOptions=Index vector (dialog)  Indices=1  OutputSizes=1
  Data Store Write27 : DataStoreWrite  DataStoreName=C2C_NMPC_Delta_DOI_H2_Weight  IndexOptions=Index vector (dialog)  Indices=1  OutputSizes=1
  Data Store Write28 : DataStoreWrite  DataStoreName=C2C_NMPC_SOOT_Weight  IndexOptions=Index vector (dialog)  Indices=1  OutputSizes=1
  Data Store Write29 : DataStoreWrite  DataStoreName=C2C_NMPC_MPRR_Weight  IndexOptions=Index vector (dialog)  Indices=1  OutputSizes=1
  Data Store Write3 : DataStoreWrite  DataStoreName=C2C_NMPC_constraints_low_DOI_H2  IndexOptions=Index vector (dialog)  Indices=1  OutputSizes=1
  Data Store Write30 : DataStoreWrite  DataStoreName=C2C_NMPC_DOI_Main_Weight  IndexOptions=Index vector (dialog)  Indices=1  OutputSizes=1
  Data Store Write31 : DataStoreWrite  DataStoreName=C2C_NMPC_P2M_Weight  IndexOptions=Index vector (dialog)  Indices=1  OutputSizes=1
  Data Store Write32 : DataStoreWrite  DataStoreName=C2C_NMPC_SOI_Main_Weight  IndexOptions=Index vector (dialog)  Indices=1  OutputSizes=1
  Data Store Write33 : DataStoreWrite  DataStoreName=C2C_NMPC_DOI_H2_Weight  IndexOptions=Index vector (dialog)  Indices=1  OutputSizes=1
  Data Store Write34 : DataStoreWrite  DataStoreName=C2C_NMPC_Delta_DOI_Main_Weight  IndexOptions=Index vector (dialog)  Indices=1  OutputSizes=1
  Data Store Write35 : DataStoreWrite  DataStoreName=C2C_NMPC_Delta_P2M_Weight  IndexOptions=Index vector (dialog)  Indices=1  OutputSizes=1
  Data Store Write36 : DataStoreWrite  DataStoreName=C2C_NMPC_alpha  IndexOptions=Index vector (dialog)  Indices=1  OutputSizes=1
  Data Store Write37 : DataStoreWrite  DataStoreName=C2C_NMPC_beta  IndexOptions=Index vector (dialog)  Indices=1  OutputSizes=1
  Data Store Write38 : DataStoreWrite  DataStoreName=C2C_NMPC_gamma  IndexOptions=Index vector (dialog)  Indices=1  OutputSizes=1
  Data Store Write39 : DataStoreWrite  DataStoreName=C2C_NMPC_constraints_low_SOOT_soft  IndexOptions=Index vector (dialog)  Indices=1  OutputSizes=1
  Data Store Write4 : DataStoreWrite  DataStoreName=C2C_NMPC_constraints_up_DOI_main  IndexOptions=Index vector (dialog)  Indices=1  OutputSizes=1
  Data Store Write40 : DataStoreWrite  DataStoreName=C2C_NMPC_constraints_low_MPRR_soft  IndexOptions=Index vector (dialog)  Indices=1  OutputSizes=1
  Data Store Write41 : DataStoreWrite  DataStoreName=C2C_NMPC_constraints_up_IMEP_soft  IndexOptions=Index vector (dialog)  Indices=1  OutputSizes=1
  Data Store Write42 : DataStoreWrite  DataStoreName=C2C_NMPC_constraints_up_NOX_soft  IndexOptions=Index vector (dialog)  Indices=1  OutputSizes=1
  Data Store Write43 : DataStoreWrite  DataStoreName=C2C_NMPC_constraints_up_SOOT_soft  IndexOptions=Index vector (dialog)  Indices=1  OutputSizes=1
  Data Store Write44 : DataStoreWrite  DataStoreName=C2C_NMPC_constraints_up_MPRR_soft  IndexOptions=Index vector (dialog)  Indices=1  OutputSizes=1
  Data Store Write45 : DataStoreWrite  DataStoreName=C2C_NMPC_constraints_low_IMEP_soft  IndexOptions=Index vector (dialog)  Indices=1  OutputSizes=1
  Data Store Write46 : DataStoreWrite  DataStoreName=C2C_NMPC_constraints_low_NOX_soft  IndexOptions=Index vector (dialog)  Indices=1  OutputSizes=1
  Data Store Write5 : DataStoreWrite  DataStoreName=C2C_NMPC_constraints_up_P2M  IndexOptions=Index vector (dialog)  Indices=1  OutputSizes=1
  Data Store Write6 : DataStoreWrite  DataStoreName=C2C_NMPC_constraints_up_SOI_main  IndexOptions=Index vector (dialog)  Indices=1  OutputSizes=1
  Data Store Write7 : DataStoreWrite  DataStoreName=C2C_NMPC_constraints_up_DOI_H2  IndexOptions=Index vector (dialog)  Indices=1  OutputSizes=1
  Data Store Write8 : DataStoreWrite  DataStoreName=C2C_NMPC_constraints_low_IMEP  IndexOptions=Index vector (dialog)  Indices=1  OutputSizes=1
  Data Store Write9 : DataStoreWrite  DataStoreName=C2C_NMPC_constraints_low_NOX  IndexOptions=Index vector (dialog)  Indices=1  OutputSizes=1
  Demux : Demux  Outputs=3
  Demux1 : Demux  Outputs=6
  Demux2 : Demux  Outputs=24
  Demux3 : Demux  Outputs=12
  Demux4 : Demux  Outputs=2
  Demux5 : Demux  Outputs=8
  Display{,1..57} (58 alike) : Display
  Gain{,1,4..5,8,17..41,43..45} (33 alike) : Gain  Gain=1e-6
  Gain{2..3,6..7,9..16,42,46} (14 alike) : Gain
  IMEP1 : Gain
  IMEP_Ref1 : Gain
  IMEP_Ref2 : Gain
  IMEP_Ref3 : Gain
  MPRR1 : Gain
  Mux1 : Mux  Inputs=8
  NOX1 : Gain  Gain=1/1e3
  Selector : Selector  IndexOptions=Index vector (dialog)  Indices=[1:6]  OutputSizes=1
  Selector1 : Selector  IndexOptions=Index vector (dialog)  Indices=[7:30]  OutputSizes=1
  Selector2 : Selector  IndexOptions=Index vector (dialog)  Indices=[31:42]  OutputSizes=1
  Selector3 : Selector  IndexOptions=Index vector (dialog)  Indices=[54]  OutputSizes=1
  Selector4 : Selector  IndexOptions=Index vector (dialog)  Indices=[43:45]  OutputSizes=1
  Selector5 : Selector  IndexOptions=Index vector (dialog)  Indices=[55:56]  OutputSizes=1
  Selector6 : Selector  IndexOptions=Index vector (dialog)  Indices=[46:53]  OutputSizes=1
  Soot1 : Gain  Gain=1/1e4
  udp_outputs : Outport
  controller_mode : Outport  Port=2
  wires:
  Demux2/16 -> Gain16/1
  Demux2/1 -> Gain/1
  Demux3/9 -> Gain33/1
  Demux2/9 -> Gain9/1
  Demux2/2 -> Gain2/1
  Demux3/11 -> Gain35/1
  Demux1/1 -> IMEP1/1
  Demux2/3 -> Gain3/1
  Demux2/23 -> Gain24/1
  Demux2/18 -> Gain18/1
  Demux3/2 -> Gain26/1
  Demux1/2 -> NOX1/1
  Demux2/12 -> Gain12/1
  Demux2/19 -> Gain19/1
  Demux2/21 -> Gain21/1
  Demux1/3 -> Soot1/1
  Demux3/3 -> Gain27/1
  Demux2/15 -> Gain15/1
  Demux2/7 -> Gain7/1
  Demux3/10 -> Gain34/1
  Demux2/10 -> Gain10/1
  Demux3/8 -> Gain32/1
  Demux2/4 -> Gain4/1
  Demux2/22 -> Gain22/1
  Demux2/13 -> Gain13/1
  Demux2/14 -> Gain14/1
  Demux2/20 -> Gain20/1
  Demux2/11 -> Gain11/1
  Demux2/5 -> Gain5/1
  Selector/1 -> Demux1/1
  Demux3/6 -> Gain30/1
  Demux2/6 -> Gain6/1
  Mux1/1 -> udp_outputs/1
  Demux2/17 -> Gain17/1
  Demux2/24 -> Gain23/1
  Demux2/8 -> Gain8/1
  Demux3/4 -> Gain28/1
  Demux1/4 -> MPRR1/1
  Demux3/7 -> Gain31/1
  Demux3/1 -> Gain25/1
  Demux1/6 -> Counter1/1
  Counter1/1 -> Display45/1, Mux1/6
  NOX1/1 -> Display48/1, Mux1/2
  Soot1/1 -> Display47/1, Mux1/3
  Demux3/12 -> Gain36/1
  Demux1/5 -> IMEP_Ref1/1
  IMEP1/1 -> Display49/1, Mux1/1
  Demux3/5 -> Gain29/1
  Add/1 -> Display1/1, Demux3/1
  Constant1/1 -> Add/2
  Gain/1 -> Display2/1, Data Store Write/1
  Gain2/1 -> Display3/1, Data Store Write1/1
  Gain3/1 -> Data Store Write2/1, Display5/1
  Gain4/1 -> Display4/1, Data Store Write3/1
  Gain5/1 -> Display6/1, Data Store Write4/1
  Gain6/1 -> Display7/1, Data Store Write5/1
  Gain7/1 -> Display8/1, Data Store Write6/1
  Gain8/1 -> Display9/1, Data Store Write7/1
  Gain9/1 -> Display10/1, Data Store Write8/1
  Gain10/1 -> Display11/1, Data Store Write9/1
  Gain11/1 -> Display12/1, Data Store Write10/1
  Gain12/1 -> Display13/1, Data Store Write11/1
  Gain13/1 -> Data Store Write12/1, Display14/1
  Gain14/1 -> Display15/1, Data Store Write13/1
  Gain15/1 -> Data Store Write14/1, Display16/1
  Gain16/1 -> Display17/1, Data Store Write15/1
  Gain17/1 -> Display18/1, Data Store Write16/1
  Gain18/1 -> Display19/1, Data Store Write17/1
  Gain19/1 -> Display20/1, Data Store Write18/1
  Gain20/1 -> Display21/1, Data Store Write19/1
  Gain21/1 -> Display22/1, Data Store Write20/1
  Gain22/1 -> Display23/1, Data Store Write21/1
  Gain23/1 -> Display25/1, Data Store Write23/1
  Gain24/1 -> Display24/1, Data Store Write22/1
  Gain25/1 -> Display26/1, Data Store Write30/1
  Gain26/1 -> Display27/1, Data Store Write31/1
  Gain27/1 -> Display28/1, Data Store Write32/1
  Gain28/1 -> Display29/1, Data Store Write33/1
  Gain29/1 -> Display30/1, Data Store Write24/1
  Gain30/1 -> Display31/1, Data Store Write25/1
  Gain31/1 -> Display32/1, Data Store Write28/1
  Gain32/1 -> Display33/1, Data Store Write29/1
  Gain33/1 -> Display34/1, Data Store Write34/1
  Gain34/1 -> Display35/1, Data Store Write35/1
  Gain35/1 -> Display36/1, Data Store Write26/1
  Gain36/1 -> Display37/1, Data Store Write27/1
  Selector2/1 -> Add/1
  Selector1/1 -> Add1/1
  Add1/1 -> Display/1, Demux2/1
  Constant2/1 -> Add1/2
  Constant3/1 -> Add2/2
  Selector3/1 -> Add2/1
  Add2/1 -> controller_mode/1, Display38/1
  Constant4/1 -> Add3/2
  Selector4/1 -> Add3/1
  Add3/1 -> Demux/1
  Demux/1 -> Gain1/1
  Demux/2 -> Gain37/1
  Demux/3 -> Gain38/1
  Gain37/1 -> Display40/1, Data Store Write37/1
  Gain1/1 -> Display39/1, Data Store Write36/1
  Gain38/1 -> Display41/1, Data Store Write38/1
  IMEP_Ref2/1 -> Display42/1, Mux1/7
  IMEP_Ref3/1 -> Display43/1, Mux1/8
  Selector5/1 -> Demux4/1
  Demux4/2 -> IMEP_Ref3/1
  Demux4/1 -> IMEP_Ref2/1
  IMEP_Ref1/1 -> Mux1/5, Display44/1
  C2C_NMPC_constraints_low_SOOT_soft/1 -> ?
  C2C_NMPC_constraints_up_SOOT_soft/1 -> ?
  C2C_NMPC_constraints_up_MPRR_soft/1 -> ?
  C2C_NMPC_constraints_low_NOX_soft/1 -> ?
  C2C_NMPC_constraints_low_MPRR_soft/1 -> ?
  C2C_NMPC_constraints_up_NOX_soft/1 -> ?
  C2C_NMPC_constraints_up_IMEP_soft/1 -> ?
  C2C_NMPC_constraints_low_IMEP_soft/1 -> ?
  Gain41/1 -> Data Store Write39/1, Display52/1
  Gain39/1 -> Data Store Write45/1, Display50/1
  Gain40/1 -> Display51/1, Data Store Write46/1
  Demux5/3 -> Gain41/1
  Demux5/2 -> Gain40/1
  Demux5/1 -> Gain39/1
  Add4/1 -> Demux5/1
  Selector6/1 -> Add4/1
  Constant5/1 -> Add4/2
  udp_data_in/1 -> Selector5/1, Selector3/1, Selector6/1, Selector4/1, Selector2/1, Selector1/1, Selector/1
  Gain43/1 -> Data Store Write42/1, Display54/1
  Gain42/1 -> Display53/1, Data Store Write41/1
  Gain44/1 -> Data Store Write43/1, Display55/1
  Gain45/1 -> Display56/1, Data Store Write40/1
  Gain46/1 -> Data Store Write44/1, Display57/1
  Demux5/4 -> Gain45/1
  Demux5/5 -> Gain42/1
  Demux5/6 -> Gain43/1
  Demux5/7 -> Gain44/1
  Demux5/8 -> Gain46/1
  MPRR1/1 -> Display46/1, Mux1/4

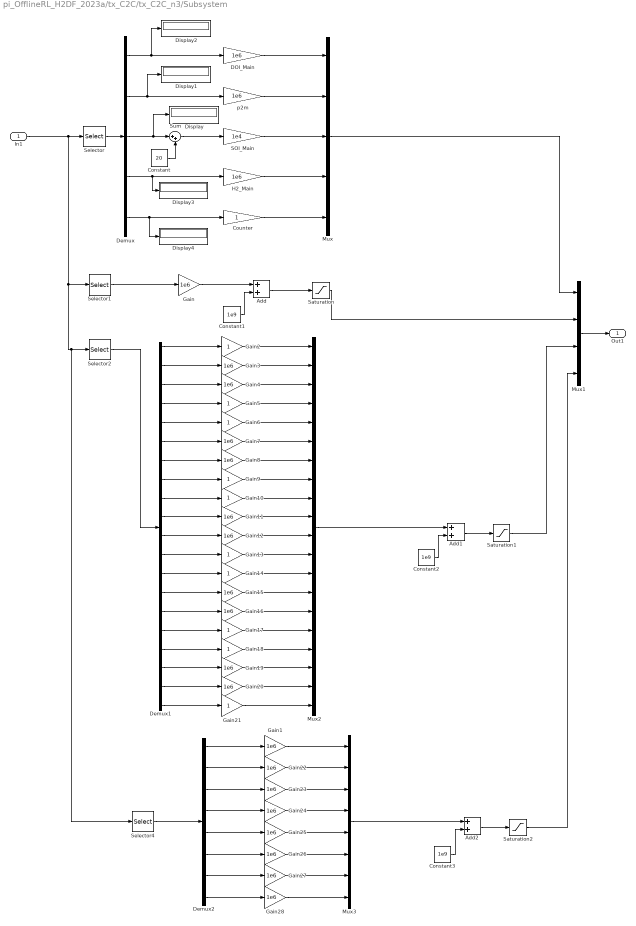
== system pi_OfflineRL_H2DF_2023a/tx_C2C/tx_C2C_n3/Subsystem ==
  In1 : Inport
  Add : Sum
  Add1 : Sum
  Add2 : Sum
  Constant : Constant  Value=20
  Constant1 : Constant  Value=1e9
  Constant2 : Constant  Value=1e9
  Constant3 : Constant  Value=1e9
  Counter : Gain
  DOI_Main : Gain  Gain=1e6
  Demux : Demux  Outputs=5
  Demux1 : Demux  Outputs=20
  Demux2 : Demux  Outputs=8
  Display{,1..4} (5 alike) : Display
  Gain{,1,3..4,7..8,11..12,15..16,19..20,22..28} (19 alike) : Gain  Gain=1e6
  Gain{2,5..6,9..10,13..14,17..18,21} (10 alike) : Gain
  H2_Main : Gain  Gain=1e6
  Mux : Mux  Inputs=5
  Mux1 : Mux
  Mux2 : Mux  Inputs=20
  Mux3 : Mux  Inputs=8
  SOI_Main : Gain  Gain=1e4
  Saturation : Saturate  UpperLimit=4e9  LowerLimit=0
  Saturation1 : Saturate  UpperLimit=4e9  LowerLimit=0
  Saturation2 : Saturate  UpperLimit=4e9  LowerLimit=0
  Selector : Selector  IndexOptions=Index vector (dialog)  Indices=[1:5]  OutputSizes=1
  Selector1 : Selector  IndexOptions=Index vector (dialog)  Indices=[6:21]  OutputSizes=1
  Selector2 : Selector  IndexOptions=Index vector (dialog)  Indices=[22:41]  OutputSizes=1
  Selector4 : Selector  IndexOptions=Index vector (dialog)  Indices=[42:49]  OutputSizes=1
  Sum : Sum  Inputs=|++
  p2m : Gain  Gain=1e6
  Out1 : Outport
  wires:
  Counter/1 -> Mux/5
  DOI_Main/1 -> Mux/1
  H2_Main/1 -> Mux/4
  SOI_Main/1 -> Mux/3
  p2m/1 -> Mux/2
  Demux/1 -> Display2/1, DOI_Main/1
  Demux/2 -> Display1/1, p2m/1
  Demux/4 -> Display3/1, H2_Main/1
  Demux/5 -> Display4/1, Counter/1
  Demux/3 -> Display/1, Sum/1
  Sum/1 -> SOI_Main/1
  Constant/1 -> Sum/2
  Selector/1 -> Demux/1
  Gain/1 -> Add/1
  Constant1/1 -> Add/2
  Selector1/1 -> Gain/1
  Mux/1 -> Mux1/1
  Mux1/1 -> Out1/1
  Add/1 -> Saturation/1
  Saturation/1 -> Mux1/2
  Saturation1/1 -> Mux1/3
  Mux2/1 -> Add1/1
  Constant2/1 -> Add1/2
  Add1/1 -> Saturation1/1
  Selector2/1 -> Demux1/1
  Demux1/1 -> Gain2/1
  Demux1/2 -> Gain3/1
  Demux1/3 -> Gain4/1
  Demux1/4 -> Gain5/1
  Demux1/5 -> Gain6/1
  Demux1/6 -> Gain7/1
  Demux1/7 -> Gain8/1
  Demux1/8 -> Gain9/1
  Demux1/9 -> Gain10/1
  Demux1/10 -> Gain11/1
  Demux1/11 -> Gain12/1
  Demux1/12 -> Gain13/1
  Demux1/13 -> Gain14/1
  Demux1/14 -> Gain15/1
  Demux1/15 -> Gain16/1
  Demux1/16 -> Gain17/1
  Demux1/17 -> Gain18/1
  Demux1/18 -> Gain19/1
  Demux1/19 -> Gain20/1
  Demux1/20 -> Gain21/1
  Gain2/1 -> Mux2/1
  Gain3/1 -> Mux2/2
  Gain4/1 -> Mux2/3
  Gain5/1 -> Mux2/4
  Gain6/1 -> Mux2/5
  Gain7/1 -> Mux2/6
  Gain8/1 -> Mux2/7
  Gain9/1 -> Mux2/8
  Gain10/1 -> Mux2/9
  Gain11/1 -> Mux2/10
  Gain12/1 -> Mux2/11
  Gain13/1 -> Mux2/12
  Gain14/1 -> Mux2/13
  Gain16/1 -> Mux2/15
  Gain15/1 -> Mux2/14
  Gain17/1 -> Mux2/16
  Gain18/1 -> Mux2/17
  Gain19/1 -> Mux2/18
  Gain20/1 -> Mux2/19
  Gain21/1 -> Mux2/20
  Gain1/1 -> Mux3/1
  Add2/1 -> Saturation2/1
  Demux2/4 -> Gain24/1
  Gain26/1 -> Mux3/6
  Demux2/5 -> Gain25/1
  In1/1 -> Selector4/1, Selector2/1, Selector1/1, Selector/1
  Gain27/1 -> Mux3/7
  Gain24/1 -> Mux3/4
  Selector4/1 -> Demux2/1
  Gain25/1 -> Mux3/5
  Demux2/3 -> Gain23/1
  Mux3/1 -> Add2/1
  Constant3/1 -> Add2/2
  Saturation2/1 -> Mux1/4
  Gain22/1 -> Mux3/2
  Gain28/1 -> Mux3/8
  Demux2/8 -> Gain28/1
  Demux2/1 -> Gain1/1
  Demux2/6 -> Gain26/1
  Demux2/7 -> Gain27/1
  Gain23/1 -> Mux3/3
  Demux2/2 -> Gain22/1

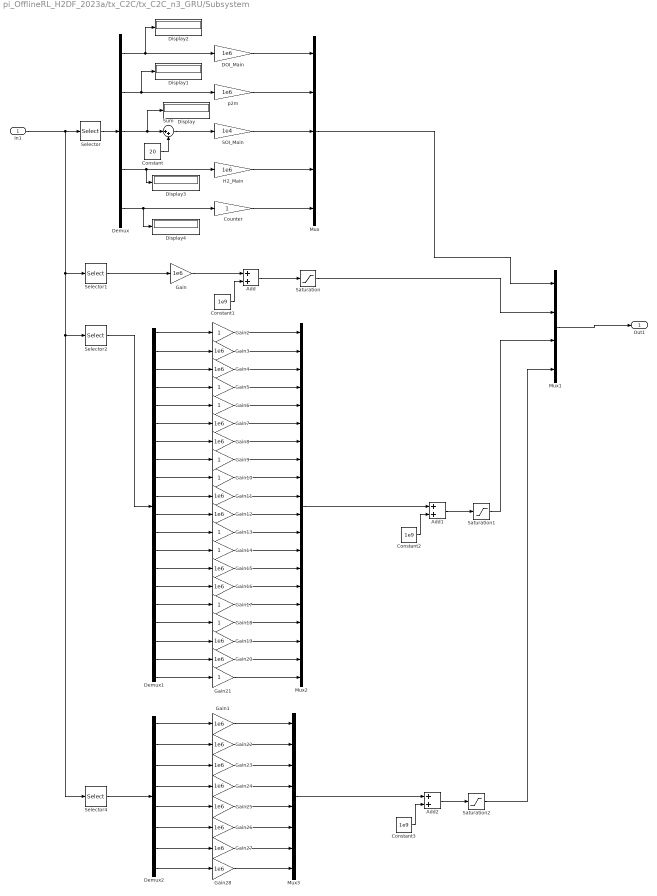
== system pi_OfflineRL_H2DF_2023a/tx_C2C/tx_C2C_n3_GRU/Subsystem ==
  In1 : Inport
  Add : Sum
  Add1 : Sum
  Add2 : Sum
  Constant : Constant  Value=20
  Constant1 : Constant  Value=1e9
  Constant2 : Constant  Value=1e9
  Constant3 : Constant  Value=1e9
  Counter : Gain
  DOI_Main : Gain  Gain=1e6
  Demux : Demux  Outputs=5
  Demux1 : Demux  Outputs=20
  Demux2 : Demux  Outputs=8
  Display{,1..4} (5 alike) : Display
  Gain{,1,3..4,7..8,11..12,15..16,19..20,22..28} (19 alike) : Gain  Gain=1e6
  Gain{2,5..6,9..10,13..14,17..18,21} (10 alike) : Gain
  H2_Main : Gain  Gain=1e6
  Mux : Mux  Inputs=5
  Mux1 : Mux
  Mux2 : Mux  Inputs=20
  Mux3 : Mux  Inputs=8
  SOI_Main : Gain  Gain=1e4
  Saturation : Saturate  UpperLimit=4e9  LowerLimit=0
  Saturation1 : Saturate  UpperLimit=4e9  LowerLimit=0
  Saturation2 : Saturate  UpperLimit=4e9  LowerLimit=0
  Selector : Selector  IndexOptions=Index vector (dialog)  Indices=[1:5]  OutputSizes=1
  Selector1 : Selector  IndexOptions=Index vector (dialog)  Indices=[6:13]  OutputSizes=1
  Selector2 : Selector  IndexOptions=Index vector (dialog)  Indices=[14:33]  OutputSizes=1
  Selector4 : Selector  IndexOptions=Index vector (dialog)  Indices=[34:41]  OutputSizes=1
  Sum : Sum  Inputs=|++
  p2m : Gain  Gain=1e6
  Out1 : Outport
  wires:
  Counter/1 -> Mux/5
  DOI_Main/1 -> Mux/1
  H2_Main/1 -> Mux/4
  SOI_Main/1 -> Mux/3
  In1/1 -> Selector4/1, Selector2/1, Selector1/1, Selector/1
  p2m/1 -> Mux/2
  Demux/1 -> Display2/1, DOI_Main/1
  Demux/2 -> Display1/1, p2m/1
  Demux/4 -> Display3/1, H2_Main/1
  Demux/5 -> Display4/1, Counter/1
  Demux/3 -> Display/1, Sum/1
  Sum/1 -> SOI_Main/1
  Constant/1 -> Sum/2
  Selector/1 -> Demux/1
  Gain/1 -> Add/1
  Constant1/1 -> Add/2
  Selector1/1 -> Gain/1
  Mux/1 -> Mux1/1
  Mux1/1 -> Out1/1
  Add/1 -> Saturation/1
  Saturation/1 -> Mux1/2
  Saturation1/1 -> Mux1/3
  Mux2/1 -> Add1/1
  Constant2/1 -> Add1/2
  Add1/1 -> Saturation1/1
  Selector2/1 -> Demux1/1
  Demux1/1 -> Gain2/1
  Demux1/2 -> Gain3/1
  Demux1/3 -> Gain4/1
  Demux1/4 -> Gain5/1
  Demux1/5 -> Gain6/1
  Demux1/6 -> Gain7/1
  Demux1/7 -> Gain8/1
  Demux1/8 -> Gain9/1
  Demux1/9 -> Gain10/1
  Demux1/10 -> Gain11/1
  Demux1/11 -> Gain12/1
  Demux1/12 -> Gain13/1
  Demux1/13 -> Gain14/1
  Demux1/14 -> Gain15/1
  Demux1/15 -> Gain16/1
  Demux1/16 -> Gain17/1
  Demux1/17 -> Gain18/1
  Demux1/18 -> Gain19/1
  Demux1/19 -> Gain20/1
  Demux1/20 -> Gain21/1
  Gain2/1 -> Mux2/1
  Gain3/1 -> Mux2/2
  Gain4/1 -> Mux2/3
  Gain5/1 -> Mux2/4
  Gain6/1 -> Mux2/5
  Gain7/1 -> Mux2/6
  Gain8/1 -> Mux2/7
  Gain9/1 -> Mux2/8
  Gain10/1 -> Mux2/9
  Gain11/1 -> Mux2/10
  Gain12/1 -> Mux2/11
  Gain13/1 -> Mux2/12
  Gain14/1 -> Mux2/13
  Gain16/1 -> Mux2/15
  Gain15/1 -> Mux2/14
  Gain17/1 -> Mux2/16
  Gain18/1 -> Mux2/17
  Gain19/1 -> Mux2/18
  Gain20/1 -> Mux2/19
  Gain21/1 -> Mux2/20
  Selector4/1 -> Demux2/1
  Demux2/1 -> Gain1/1
  Demux2/2 -> Gain22/1
  Demux2/3 -> Gain23/1
  Demux2/4 -> Gain24/1
  Gain1/1 -> Mux3/1
  Gain22/1 -> Mux3/2
  Gain23/1 -> Mux3/3
  Gain24/1 -> Mux3/4
  Saturation2/1 -> Mux1/4
  Mux3/1 -> Add2/1
  Constant3/1 -> Add2/2
  Add2/1 -> Saturation2/1
  Demux2/5 -> Gain25/1
  Demux2/6 -> Gain26/1
  Demux2/7 -> Gain27/1
  Demux2/8 -> Gain28/1
  Gain25/1 -> Mux3/5
  Gain26/1 -> Mux3/6
  Gain27/1 -> Mux3/7
  Gain28/1 -> Mux3/8

== system pi_OfflineRL_H2DF_2023a/main_C2C/main_C2C_RL/RL_Controller/Denorm_plant_IMEP_ref ==
  In : Inport
  Constant : Constant  Value=C2C_NMPC.Normalization.outputs.mean(1)
  Gain : Gain  Gain=C2C_NMPC.Normalization.outputs.std(1)
  Sum6 : Sum  Inputs=|++
  RefIn : Outport
  wires:
  In/1 -> Gain/1  "IMEP"
  Sum6/1 -> RefIn/1
  Gain/1 -> Sum6/1
  Constant/1 -> Sum6/2

== system pi_OfflineRL_H2DF_2023a/main_C2C/main_C2C_RL/RL_Controller/Denorm_plant_IMEP_ref1 ==
  In : Inport
  Constant : Constant  Value=C2C_NMPC.Normalization.outputs.mean(1)
  Gain : Gain  Gain=C2C_NMPC.Normalization.outputs.std(1)
  Sum6 : Sum  Inputs=|++
  RefIn : Outport
  wires:
  Constant/1 -> Sum6/2
  Gain/1 -> Sum6/1
  Sum6/1 -> RefIn/1
  In/1 -> Gain/1  "IMEP"

== system pi_OfflineRL_H2DF_2023a/main_C2C/main_C2C_RL/RL_Controller/RL_Controller_ifAction ==
  SelectorIn : Inport
  Observation : Inport  Port=2
  Display1 : Display
  Display6 : Display
  Merge : Merge  Inputs=3
  RL_Controller_PPO : Subsystem  Commented=on  VariantControl=fb_LSTM_321_syn
  RL_Controller_PPO1 : Subsystem  Commented=on  VariantControl=fb_LSTM_321_syn
  RL_Controller_TD3 : Subsystem  VariantControl=fb_LSTM_321_syn
  Switch Case : SwitchCase  CaseConditions={1,2,3}  ShowDefaultCase=off
  ControlsOut : Outport
  wires:
  SelectorIn/1 -> Switch Case/1
  Merge/1 -> Display1/1, ControlsOut/1
  RL_Controller_TD3/1(Control_norm_NN_params) -> Merge/1
  RL_Controller_PPO/1(Control_norm_NN_params) -> Merge/2
  Switch Case/1 -> RL_Controller_TD3/Action
  Observation/1 -> RL_Controller_PPO/1(Obs), RL_Controller_PPO1/1(Obs), RL_Controller_TD3/1(Obs)
  Switch Case/2 -> RL_Controller_PPO/Action
  Switch Case/3 -> RL_Controller_PPO1/Action
  RL_Controller_PPO1/1(Control_norm_NN_params) -> Merge/3

== system pi_OfflineRL_H2DF_2023a/main_C2C/main_C2C_RL/RL_Controller/SafetySaturation ==
  controls_nn_in : Inport
  Saturation4 : Saturate  UpperLimit=UpperLimit  LowerLimit=LowerLimit
  controls_nn_out : Outport
  wires:
  controls_nn_in/1 -> Saturation4/1
  Saturation4/1 -> controls_nn_out/1

== system pi_OfflineRL_H2DF_2023a/main_C2C/main_C2C_RL/RL_Controller/State_Augmentation ==
  controls : Inport
  Delay1 : Delay  DelayLength=1  InitialCondition=C2C_NMPC.x0(1:C2C_NMPC.Dims.n_LSTM_states)
  Delay3 : Delay  DelayLength=1  InitialCondition=C2C_NMPC.x0
  Delay4 : Delay  DelayLength=1  InitialCondition=C2C_NMPC.x0((C2C_NMPC.Dims.n_states - C2C_NMPC.Dims.n_outputs + 1):C2C_NMPC.Dims.n_states)
  Denorm_plant_IMEP_ref1 : Subsystem
  Display1 : Display
  Mux2 : Mux  Inputs=2
  Mux3 : Mux  Inputs=2
  Selector1 : Selector  IndexOptions=Index vector (dialog)  Indices=[(C2C_NMPC.Dims.n_states - C2C_NMPC.Dims.n_outputs + 1):C2C_NMPC.Dims.n_states]  OutputSizes=1
  Selector3 : Selector  IndexOptions=Index vector (dialog)  Indices=[1]  OutputSizes=1
  dyn_H2DF : Subsystem
  dyn_H2DF_state_augmentation : Subsystem
  LSTM_states : Outport
  wires:
  Delay3/1 -> Selector1/1
  Delay1/1 -> dyn_H2DF/3(last_LSTM_states), dyn_H2DF_state_augmentation/1(last_LSTM_states)
  dyn_H2DF_state_augmentation/1(LSTM_states) -> LSTM_states/1, Delay1/1, Mux3/1
  Mux2/1 -> Mux3/2
  controls/1 -> dyn_H2DF/1(controls), [controls]
  Selector1/1 -> dyn_H2DF/2(last_outputs)
  [controls] -> dyn_H2DF_state_augmentation/2(controls), Mux2/1
  Delay4/1 -> dyn_H2DF_state_augmentation/3(last_outputs)
  Mux3/1 -> Delay3/1
  Denorm_plant_IMEP_ref1/1(RefIn) -> Display1/1
  Selector3/1 -> Denorm_plant_IMEP_ref1/1(outputs)
  dyn_H2DF/1(outputs) -> Selector3/1, Delay4/1, Mux2/2
